simulink model "bus_14_take_1"  (Simulink 10.3)
settings: Solver=ode45  StartTime=0.0  StopTime=2  RelTol=1e-3
undefined symbols (not defined in the file): Discrete, linsys1, Time
libraries: spsThreePhaseVIMeasurementLib x46, spsThreePhasePISectionLineLib x20, spsThreePhaseSeriesRLCLoadLib x14, spsPMUPLLBasedPositiveSequenceLib x9, eePMU x5, spsThreePhaseTransformerTwoWindingsLib x5, spsPLLLib x4, ctrlSharedLib x3, spsSynchronousMachinepuStandardLib x3, spsThreePhaseParallelRLCLoadLib x3, spsThreePhaseBreakerLib x3, spsExcitationSystemLib x3
(part 1 of 2)
settings Model: Creator=User  LastModifiedBy=User
settings SolverCC: AlgebraicLoopSolver=Auto
settings DataIOCC: SaveFormat=Structure  SignalLoggingSaveFormat=Dataset  SaveOutput=off  SignalLogging=off  DSMLogging=off  SaveTime=off  ReturnWorkspaceOutputs=on  LoggingToFile=on
settings OptimizationCC: ExpressionDepthLimit=128  LifeSpan=auto  UseRowMajorAlgorithm=on
settings DebuggingCC: UnderspecifiedInitializationDetection=Simplified  MergeDetectMultiDrivingBlocksExec=error  FcnCallInpInsideContextMsg=error  StateNameClashWarn=none  SFUnexpectedBacktrackingDiag=error  SFNoUnconditionalDefaultTransitionDiag=error  SFExecutionAtInitializationDiag=warning  SFMachineParentedDataDiag=error  ArithmeticOperatorsInVariantConditions=error
settings HardwareCC: ProdBitPerPointer=64  ProdBitPerSizeT=64  ProdBitPerPtrDiffT=64  ProdLargestAtomicFloat=Float  ProdIntDivRoundTo=Zero  ProdEndianess=LittleEndian  ProdWordSize=64  ProdHWDeviceType=Intel->x86-64 (Windows64)
settings ModelReferenceCC: PropagateSignalLabelsOutOfModel=on
settings SFSimCC: SimUseLocalCustomCode=on  CustomCodeUndefinedFunction=FilterOut
settings RTWCC: RTWUseLocalCustomCode=on
settings CodeAppCC: StateflowObjectComments=off
settings GRTTargetCC: TargetLangStandard=C99 (ISO)  CombineOutputUpdateFcns=on  GRTInterface=off
settings ConfigComp: CovMetricSettings=dwe  CovSaveCumulativeToWorkspaceVar=off  CovSaveSingleToWorkspaceVar=off  CovExternalEMLEnable=on

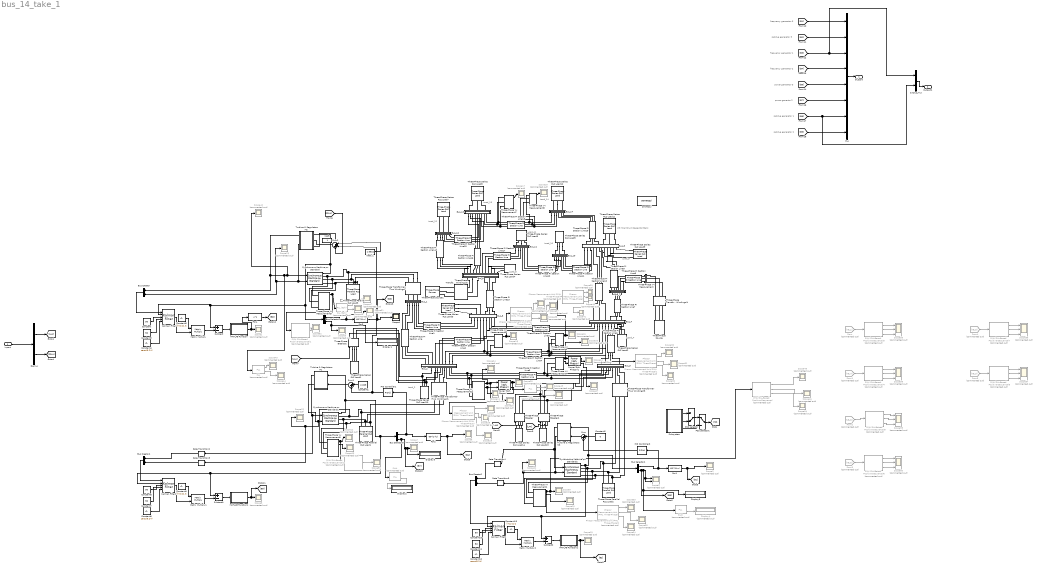
== system bus_14_take_1 ==
  note: residue generator 2
  note: residue generator 1
  note: power genertor 2
  note: power generator 3
  note: frequency generator 2
  note: frequency generator 1
  note: residue generator 3
  note: frequency generator 3
  note: Load_2
  note: Load_10
  note: Load_13
  note: Load_12
  note: 25 MVar Shunt
      | Capacitor Bank
  note: Load_9
  note: Load_11
  note: Load_6
  note: Load_4
  note: Load_14
  note: Load_5
  Inport : Inport
  Bus Creator : BusCreator  Inputs=2
  Bus Creator1 : BusCreator  Inputs=2
  Bus Creator2 : BusCreator  Inputs=2
  Bus Selector1 : BusSelector  OutputSignals="Mechanical.Rotor speed deviation  dw (pu),Mechanical.Electrical power  Pe (pu)"
  Bus Selector2 : BusSelector  OutputSignals="Mechanical.Rotor speed deviation  dw (pu),Mechanical.Electrical power  Pe (pu)"
  Bus Selector3 : BusSelector  OutputSignals="Mechanical.Rotor speed deviation  dw (pu),Mechanical.Electrical power  Pe (pu)"
  Bus_1 : Subsystem
  Bus_10 : Subsystem
  Bus_11 : Subsystem
  Bus_12 : Subsystem
  Bus_13 : Subsystem
  Bus_14 : Subsystem
  Bus_2 : Subsystem
  Bus_3 : Subsystem
  Bus_4 : Subsystem
  Bus_5 : Subsystem
  Bus_6 : Subsystem
  Bus_7 : Subsystem
  Bus_9 : Subsystem
  Constant{,3,6..7,10..11} (6 alike) : Constant  Value=50
  Constant1 : Constant  Value=2.009
  Constant12 : Constant  Value=zeros(8,24)
  Constant13 : Constant  Value=linsys1.C
  Constant2 : Constant  Value=0
  Constant4 : Constant  Value=zeros(8,24)
  Constant5 : Constant  Value=linsys1.C
  Constant8 : Constant  Value=zeros(8,24)
  Constant9 : Constant  Value=linsys1.C
  Demux : Demux  Outputs=2
  Display{1..3,5} (4 alike) : Display
  Display4 : Display  Commented=on
  Fcn1 : Fcn  Expr=60*(1+u)
  Fcn2 : Fcn  Expr=60*(1+u)
  Fcn3 : Fcn  Expr=60*(1+u)
  Fcn4 : Fcn  Expr=u*1
  From : From  Commented=on  GotoTag=VB_2  TagVisibility=global
  From1 : From  Commented=on  GotoTag=VB_4  TagVisibility=global
  From2 : From  Commented=on  GotoTag=VB_5  TagVisibility=global
  From3 : From  Commented=on  GotoTag=VB_6  TagVisibility=global
  From4 : From  Commented=on  GotoTag=VB_8  TagVisibility=global
  From5 : From  Commented=on  GotoTag=VB_9  TagVisibility=global
  Kalman Filter : ctrlSharedLib/Kalman Filter  TimeDomain=Discrete-Time  UseCurrentEstimator=on  ModelSource=Individual A, B, C, D matrices  ModelSourceVariable=ss(0.95,1,1,0,1)  A=linsys1.A  B=linsys1.B  C=linsys1.C  D=linsys1.D  NumberOfStates=1  NumberOfInputs=1  NumberOfOutputs=1  InitialEstimateSource=Dialog  X0=0  P0=10  UseK=off  UseGH=off  NumberOfProcessNoiseInputs=1  G=1  TimeInvariantG=on  H=0  TimeInvariantH=on  Q=0.05  TimeInvariantQ=off  R=1  TimeInvariantR=off  N=0  TimeInvariantN=off  AddInputPort=on  AddEnablePort=off  OutputEstimatedY=off  OutputP=off  Ts=-1
  Kalman Filter1 : ctrlSharedLib/Kalman Filter  TimeDomain=Discrete-Time  UseCurrentEstimator=on  ModelSource=Individual A, B, C, D matrices  ModelSourceVariable=ss(0.95,1,1,0,1)  A=linsys1.A  B=linsys1.B  C=linsys1.C  D=linsys1.D  NumberOfStates=1  NumberOfInputs=1  NumberOfOutputs=1  InitialEstimateSource=Dialog  X0=0  P0=10  UseK=off  UseGH=off  NumberOfProcessNoiseInputs=1  G=1  TimeInvariantG=on  H=0  TimeInvariantH=on  Q=0.05  TimeInvariantQ=off  R=1  TimeInvariantR=off  N=0  TimeInvariantN=off  AddInputPort=on  AddEnablePort=off  OutputEstimatedY=off  OutputP=off  Ts=-1
  Kalman Filter2 : ctrlSharedLib/Kalman Filter  TimeDomain=Discrete-Time  UseCurrentEstimator=on  ModelSource=Individual A, B, C, D matrices  ModelSourceVariable=ss(0.95,1,1,0,1)  A=linsys1.A  B=linsys1.B  C=linsys1.C  D=linsys1.D  NumberOfStates=1  NumberOfInputs=1  NumberOfOutputs=1  InitialEstimateSource=Dialog  X0=0  P0=10  UseK=off  UseGH=off  NumberOfProcessNoiseInputs=1  G=1  TimeInvariantG=on  H=0  TimeInvariantH=on  Q=0.05  TimeInvariantQ=off  R=1  TimeInvariantR=off  N=0  TimeInvariantN=off  AddInputPort=on  AddEnablePort=off  OutputEstimatedY=off  OutputP=off  Ts=-1
  MATLAB Function : MATLAB Function  TreatAsAtomicUnit=on
  MATLAB Function1 : MATLAB Function  TreatAsAtomicUnit=on
  MATLAB Function2 : MATLAB Function  TreatAsAtomicUnit=on
  Matrix Multiply : Product  Multiplication=Matrix(*)
  Matrix Multiply1 : Product  Multiplication=Matrix(*)
  Matrix Multiply2 : Product  Multiplication=Matrix(*)
  Mux : Mux  Inputs=8
  PID Controller1 : pid_lib/PID Controller  Controller=PID  Form=Parallel  TimeDomain=Discrete-time  UseExternalTs=off  SampleTime=-1  IntegratorMethod=Forward Euler  FilterMethod=Forward Euler  ControllerParametersSource=internal  P=-2.009  I=10  D=0  UseFilter=on  N=100  TunerSelectOption=Frequency Response Based  InitialConditionSource=internal  InitialConditionForIntegrator=0  InitialConditionForFilter=0  DifferentiatorICPrevScaledInput=0  ExternalReset=none  TrackingMode=off  Kt=1  LimitOutput=off  SatLimitsSource=internal  UpperSaturationLimit=inf  LowerSaturationLimit=-inf  LinearizeAsGain=on  AntiWindupMode=none  Kb=1  POutMin=[]  POutMax=[]  IOutMin=[]  IOutMax=[]  DOutMin=[]  DOutMax=[]  NOutMin=[]  NOutMax=[]  SumOutMin=[]  SumOutMax=[]  SaturationOutMin=[]  SaturationOutMax=[]  PParamMin=[]  PParamMax=[]  IParamMin=[]  IParamMax=[]  DParamMin=[]  DParamMax=[]  NParamMin=[]  NParamMax=[]  KbParamMin=[]  KbParamMax=[]  KtParamMin=[]  KtParamMax=[]  KbOutMin=[]  KbOutMax=[]  KtOutMin=[]  KtOutMax=[]  IntegratorOutMin=[]  IntegratorOutMax=[]  FilterOutMin=[]  FilterOutMax=[]  SumI1OutMin=[]  SumI1OutMax=[]  SumI2OutMin=[]  SumI2OutMax=[]  SumI3OutMin=[]  SumI3OutMax=[]  SumI4OutMin=[]  SumI4OutMax=[]  SumDOutMin=[]  SumDOutMax=[]  DifferentiatorOutMin=[]  DifferentiatorOutMax=[]  FilterDiffOutCoefMin=[]  FilterDiffOutCoefMax=[]  ReciprocalOutMin=[]  ReciprocalOutMax=[]  SumDenOutMin=[]  SumDenOutMax=[]  SumNumOutMin=[]  SumNumOutMax=[]  DivideOutMin=[]  DivideOutMax=[]  UdiffTsProdOutMin=[]  UdiffTsProdOutMax=[]  NTsProdOutMin=[]  NTsProdOutMax=[]  UintegralTsProdOutMin=[]  UintegralTsProdOutMax=[]  UngainTsProdOutMin=[]  UngainTsProdOutMax=[]  IntegratorContinuousStateAttributes=''  IntegratorStateMustResolveToSignalObject=off  IntegratorRTWStateStorageClass=Auto  FilterContinuousStateAttributes=''  FilterStateMustResolveToSignalObject=off  FilterRTWStateStorageClass=Auto  ParallelPVariant=InternalParameters  IdealPVariant=Disabled  IVariant=InternalParameters  DVariant=InternalParameters  IntegratorVariant=Discrete  SatVariant=Disabled  AWVariant=Passthrough  PCopyVariant=Disabled  TRVariant=Disabled  FdbkBlocksVariant=Forward  IdealPFdbkVariant=Disabled  SatFdbkVariant=Disabled  DerivativeFilterVariant=ForwardEulerFilter  NVariant=InternalParameters  NCopyVariant=Disabled  FilterICVariant=InternalICsFilter  IntegratorICVariant=InternalICs  ExternalResetVariant=Disabled  TRSumVariant=Passthrough  SumFdbkVariant=Disabled  SumVariant=Sum_PID  TsampFilterVariant=InternalTs  TsampNgainVariant=Passthrough  TsampIntegralVariant=Passthrough  ExternalSaturationOutDataTypeStr=Inherit: Same as second input
  PID Controller2 : pid_lib/PID Controller  Controller=PID  Form=Parallel  TimeDomain=Discrete-time  UseExternalTs=off  SampleTime=-1  IntegratorMethod=Forward Euler  FilterMethod=Forward Euler  ControllerParametersSource=internal  P=-2  I=10  D=0  UseFilter=on  N=100  TunerSelectOption=Transfer Function Based (PID Tuner App)  InitialConditionSource=internal  InitialConditionForIntegrator=0  InitialConditionForFilter=0  DifferentiatorICPrevScaledInput=0  ExternalReset=none  TrackingMode=off  Kt=1  LimitOutput=off  SatLimitsSource=internal  UpperSaturationLimit=inf  LowerSaturationLimit=-inf  LinearizeAsGain=on  AntiWindupMode=none  Kb=1  POutMin=[]  POutMax=[]  IOutMin=[]  IOutMax=[]  DOutMin=[]  DOutMax=[]  NOutMin=[]  NOutMax=[]  SumOutMin=[]  SumOutMax=[]  SaturationOutMin=[]  SaturationOutMax=[]  PParamMin=[]  PParamMax=[]  IParamMin=[]  IParamMax=[]  DParamMin=[]  DParamMax=[]  NParamMin=[]  NParamMax=[]  KbParamMin=[]  KbParamMax=[]  KtParamMin=[]  KtParamMax=[]  KbOutMin=[]  KbOutMax=[]  KtOutMin=[]  KtOutMax=[]  IntegratorOutMin=[]  IntegratorOutMax=[]  FilterOutMin=[]  FilterOutMax=[]  SumI1OutMin=[]  SumI1OutMax=[]  SumI2OutMin=[]  SumI2OutMax=[]  SumI3OutMin=[]  SumI3OutMax=[]  SumI4OutMin=[]  SumI4OutMax=[]  SumDOutMin=[]  SumDOutMax=[]  DifferentiatorOutMin=[]  DifferentiatorOutMax=[]  FilterDiffOutCoefMin=[]  FilterDiffOutCoefMax=[]  ReciprocalOutMin=[]  ReciprocalOutMax=[]  SumDenOutMin=[]  SumDenOutMax=[]  SumNumOutMin=[]  SumNumOutMax=[]  DivideOutMin=[]  DivideOutMax=[]  UdiffTsProdOutMin=[]  UdiffTsProdOutMax=[]  NTsProdOutMin=[]  NTsProdOutMax=[]  UintegralTsProdOutMin=[]  UintegralTsProdOutMax=[]  UngainTsProdOutMin=[]  UngainTsProdOutMax=[]  IntegratorContinuousStateAttributes=''  IntegratorStateMustResolveToSignalObject=off  IntegratorRTWStateStorageClass=Auto  FilterContinuousStateAttributes=''  FilterStateMustResolveToSignalObject=off  FilterRTWStateStorageClass=Auto  ParallelPVariant=InternalParameters  IdealPVariant=Disabled  IVariant=InternalParameters  DVariant=InternalParameters  IntegratorVariant=Discrete  SatVariant=Disabled  AWVariant=Passthrough  PCopyVariant=Disabled  TRVariant=Disabled  FdbkBlocksVariant=Forward  IdealPFdbkVariant=Disabled  SatFdbkVariant=Disabled  DerivativeFilterVariant=ForwardEulerFilter  NVariant=InternalParameters  NCopyVariant=Disabled  FilterICVariant=InternalICsFilter  IntegratorICVariant=InternalICs  ExternalResetVariant=Disabled  TRSumVariant=Passthrough  SumFdbkVariant=Disabled  SumVariant=Sum_PID  TsampFilterVariant=InternalTs  TsampNgainVariant=Passthrough  TsampIntegralVariant=Passthrough  ExternalSaturationOutDataTypeStr=Inherit: Same as second input
  PLL{,2,4..5} (4 alike) : spsPLLLib/PLL  Commented=on  Fmin=45  Par_Init=[0, 60]  ParK=[180, 3200, 1]  TcD=1e-4  MaxRateChangeFreq=12  FilterCutOffFreq=25  Ts=0  AGC=on
      settings: SourceProductBaseCode=PS
  PLL (3ph) : spsPLL3phLib/PLL (3ph)  Commented=on  Fmin=45  Par_Init=[0, 60]  ParK=[180, 3200, 1]  TcD=1e-4  MaxRateChangeFreq=12  FilterCutOffFreq=25  Ts=0  AGC=on
  PMU (PLL-Based, Positive-Sequence){,1..8} (9 alike) : spsPMUPLLBasedPositiveSequenceLib/PMU (PLL-Based, Positive-Sequence)  Commented=on  nominalFrequency=60  samplingRate=64  reportingFactor=1
      settings: SourceProductBaseCode=PS
  PSS selector : ManualSwitch  CurrentSetting=0
  PSS selector1 : ManualSwitch
  Phasor Measurement Unit (PMU, Three-Phase){,1..4} (5 alike) : eePMU/Phasor Measurement Unit (PMU, Three-Phase)  Commented=on  frequency=60  Nsr=64  k=1
      settings: SourceProductBaseCode=PS
  "Power (3ph, Phasor)" : spsPower3phPhasorLib/Power (3ph, Phasor)
      settings: SourceProductBaseCode=PS
  "Power (3ph, Phasor)1" : spsPower3phPhasorLib/Power (3ph, Phasor)
      settings: SourceProductBaseCode=PS
  Rate Transition{2..5} (4 alike) : RateTransition
  Scope{,1..2,5..54} (53 alike) : Scope  Commented=on
  Scope3 : Scope  Commented=on  NumInputPorts=2
  Scope4 : Scope
  Scope{55..60} (6 alike) : Scope  Commented=on  NumInputPorts=3
  Subsystem : Subsystem
  Subtract : Sum  Inputs=+-
  Subtract1 : Sum  Inputs=+-
  Subtract2 : Sum  Inputs=+-
  Sum : Sum  Inputs=|++
  Sum1 : Sum  Inputs=|++
  Sum2 : Sum  Inputs=|++-
  Synchronous Machine pu Standard : spsSynchronousMachinepuStandardLib/Synchronous Machine pu Standard  PresetModel=No  MechanicalLoad=Mechanical power Pm  ShowDetailedParameters=on  RotorType=Salient-pole  Units=per unit standard parameters  MeasurementBus=off  NominalParameters="[90E6  146280   60 ]"  Reactances1=[ 1.81, 0.3, 0.23, 1.76, 0.65, 0.25, 0.15 ]  Reactances2=[ 1.305, 0.296, 0.252, 0.474, 0.243, 0.18 ]  dAxisTimeConstants=Short-circuit  qAxisTimeConstants=Open-circuit  TimeConstants1="[ 4.4849  0.0681  0.1  ]"  TimeConstants2=[ 8.0, 0.03, 1.0, 0.07 ]  TimeConstants3="[  4.49  0.0681  0.0513  ]"  TimeConstants4=[ 8.0, 0.03, 0.3371, 0.0295 ]  TimeConstants5=[ 1.01, 0.053, 0.1 ]  TimeConstants6=[ 1.3201, 0.023, 1.0, 0.07 ]  TimeConstants7=[0.012 0.003 0.003]  TimeConstants8=[ 1.3201, 0.0231, 0.3371, 0.0295 ]  StatorResistance=2.8544e-3  Mechanical="[ 3.7 0  32]"  PolePairs=20  InitialConditions=[0 -55.1684 1.72023 1.72023 1.72023 -10.3587 -130.359 109.641 2.41694]  SetSaturation=off  Saturation=[0.6404,0.7127,0.8441,0.9214,0.9956,1.082,1.19,1.316,1.457;0.7,0.7698,0.8872,0.9466,0.9969,1.046,1.1,1.151,1.201]  LoadFlowParameters=[1 0 0 0 0]  TsPowergui=0  TsBlock=-1  IterativeModel=Trapezoidal non iterative  IterativeDiscreteModel=Trapezoidal non iterative  BusType=swing  Pref=0  Qref=0  Qmin=-inf  Qmax=inf  PLF=0  QLF=0
      settings: SourceProductBaseCode=PS
  Synchronous Machine pu Standard1 : spsSynchronousMachinepuStandardLib/Synchronous Machine pu Standard  PresetModel=No  MechanicalLoad=Mechanical power Pm  ShowDetailedParameters=on  RotorType=Salient-pole  Units=per unit standard parameters  MeasurementBus=off  NominalParameters="[90E6  144210   60 ]"  Reactances1=[ 1.81, 0.3, 0.23, 1.76, 0.65, 0.25, 0.15 ]  Reactances2=[ 1.305, 0.296, 0.252, 0.474, 0.243, 0.18 ]  dAxisTimeConstants=Short-circuit  qAxisTimeConstants=Open-circuit  TimeConstants1="[ 4.4849  0.0681  0.1  ]"  TimeConstants2=[ 8.0, 0.03, 1.0, 0.07 ]  TimeConstants3="[  4.49  0.0681  0.0513  ]"  TimeConstants4=[ 8.0, 0.03, 0.3371, 0.0295 ]  TimeConstants5=[ 1.01, 0.053, 0.1 ]  TimeConstants6=[ 1.3201, 0.023, 1.0, 0.07 ]  TimeConstants7=[0.012 0.003 0.003]  TimeConstants8=[ 1.3201, 0.0231, 0.3371, 0.0295 ]  StatorResistance=2.8544e-3  Mechanical="[ 3.7 0  32]"  PolePairs=20  InitialConditions=[0 -52.2742 2.06355 2.06355 2.06355 -13.2061 -133.206 106.794 2.88545]  SetSaturation=off  Saturation=[0.6404,0.7127,0.8441,0.9214,0.9956,1.082,1.19,1.316,1.457;0.7,0.7698,0.8872,0.9466,0.9969,1.046,1.1,1.151,1.201]  LoadFlowParameters=[1,0,0,0,0]  TsPowergui=0  TsBlock=-1  IterativeModel=Trapezoidal non iterative  IterativeDiscreteModel=Trapezoidal non iterative  BusType=PV  Pref=0  Qref=0  Qmin=-inf  Qmax=inf  PLF=0  QLF=0
      settings: SourceProductBaseCode=PS
  Synchronous Machine pu Standard2 : spsSynchronousMachinepuStandardLib/Synchronous Machine pu Standard  PresetModel=No  MechanicalLoad=Mechanical power Pm  ShowDetailedParameters=on  RotorType=Salient-pole  Units=per unit standard parameters  MeasurementBus=off  NominalParameters="[90E6  139380  60 ]"  Reactances1=[ 1.81, 0.3, 0.23, 1.76, 0.65, 0.25, 0.15 ]  Reactances2=[ 1.305, 0.296, 0.252, 0.474, 0.243, 0.18 ]  dAxisTimeConstants=Short-circuit  qAxisTimeConstants=Open-circuit  TimeConstants1="[ 4.4849  0.0681  0.1  ]"  TimeConstants2=[ 8.0, 0.03, 1.0, 0.07 ]  TimeConstants3="[  4.49  0.0681  0.0513  ]"  TimeConstants4=[ 8.0, 0.03, 0.3371, 0.0295 ]  TimeConstants5=[ 1.01, 0.053, 0.1 ]  TimeConstants6=[ 1.3201, 0.023, 1.0, 0.07 ]  TimeConstants7=[0.012 0.003 0.003]  TimeConstants8=[ 1.3201, 0.0231, 0.3371, 0.0295 ]  StatorResistance=2.8544e-3  Mechanical="[ 3.7 0  32]"  PolePairs=20  InitialConditions=[0 -114.329 0.550177 0.550177 0.550177 -114.259 -234.259 5.74123 1.7297]  SetSaturation=off  Saturation=[0.6404,0.7127,0.8441,0.9214,0.9956,1.082,1.19,1.316,1.457;0.7,0.7698,0.8872,0.9466,0.9969,1.046,1.1,1.151,1.201]  LoadFlowParameters=[1,0,0,0,0]  TsPowergui=0  TsBlock=-1  IterativeModel=Trapezoidal non iterative  IterativeDiscreteModel=Trapezoidal non iterative  BusType=PV  Pref=0  Qref=0  Qmin=50096006  Qmax=50096006  PLF=0  QLF=0
      settings: SourceProductBaseCode=PS
  Three-Phase PI Section Line : spsThreePhasePISectionLineLib/Three-Phase PI Section Line  LConnTagsString=a|b|c  RConnTagsString=A|B|C  Length=44.47  Frequency=60  Resistances=[ 0.1921 0.5763]  Inductances=[ 0.0016 0.0047]  Capacitances=[7.14e-9 2.14e-8]
  Three-Phase PI Section Line1 : spsThreePhasePISectionLineLib/Three-Phase PI Section Line  LConnTagsString=a|b|c  RConnTagsString=A|B|C  Length=78.64  Frequency=60  Resistances=[ 0.3029 0.9086]  Inductances=[ 0.0033 0.0099]  Capacitances=[3.35e-9 1.01e-8]
  Three-Phase PI Section Line10 : spsThreePhasePISectionLineLib/Three-Phase PI Section Line  LConnTagsString=a|b|c  RConnTagsString=A|B|C  Length=8.39  Frequency=60  Resistances=[ 0.0001 0.0003]  Inductances=[ 0.0775 0.2325]  Capacitances=[1.43e-10 4.3e-10]
  Three-Phase PI Section Line11 : spsThreePhasePISectionLineLib/Three-Phase PI Section Line  LConnTagsString=a|b|c  RConnTagsString=A|B|C  Length=3.27  Frequency=60  Resistances=[ 0.2144 0.6431]  Inductances=[ 0.0015 0.0045]  Capacitances=[1.84e-11 5.52e-11]
  Three-Phase PI Section Line12 : spsThreePhasePISectionLineLib/Three-Phase PI Section Line  LConnTagsString=a|b|c  RConnTagsString=A|B|C  Length=4.93  Frequency=60  Resistances=[ 0.3667 1.1002]  Inductances=[ 0.0023 0.0068]  Capacitances=[1.22e-11 3.66e-11]
  Three-Phase PI Section Line13 : spsThreePhasePISectionLineLib/Three-Phase PI Section Line  LConnTagsString=a|b|c  RConnTagsString=A|B|C  Length=5.65  Frequency=60  Resistances=[ 0.0001 0.0003]  Inductances=[ 0.0522 0.1565]  Capacitances=[2.13e-10 6.39e-10]
  Three-Phase PI Section Line14 : spsThreePhasePISectionLineLib/Three-Phase PI Section Line  LConnTagsString=a|b|c  RConnTagsString=A|B|C  Length=5.69  Frequency=60  Resistances=[ 0.4760 1.4281]  Inductances=[ 0.0026 0.0079]  Capacitances=[1.06e-11 3.17e-11]
  Three-Phase PI Section Line15 : spsThreePhasePISectionLineLib/Three-Phase PI Section Line  LConnTagsString=a|b|c  RConnTagsString=A|B|C  Length=5.03  Frequency=60  Resistances=[ 0.9679 2.9038]  Inductances=[ 0.0023 0.0070]  Capacitances=[1.20e-11 3.59e-11]
  Three-Phase PI Section Line16 : spsThreePhasePISectionLineLib/Three-Phase PI Section Line  LConnTagsString=a|b|c  RConnTagsString=A|B|C  Length=4.06  Frequency=60  Resistances=[ 0.3590 1.0770]  Inductances=[ 0.0019 0.0056]  Capacitances=[1.48e-11 4.44e-11]
  Three-Phase PI Section Line17 : spsThreePhasePISectionLineLib/Three-Phase PI Section Line  LConnTagsString=a|b|c  RConnTagsString=A|B|C  Length=5.02  Frequency=60  Resistances=[ 0.4172 1.2515]  Inductances=[ 0.0023 0.0070]  Capacitances=[1.20e-11 3.60e-11]
  Three-Phase PI Section Line18 : spsThreePhasePISectionLineLib/Three-Phase PI Section Line  LConnTagsString=a|b|c  RConnTagsString=A|B|C  Length=6.64  Frequency=60  Resistances=[ 0.5676 1.7027]  Inductances=[ 0.0031 0.0092]  Capacitances=[9.06e-12 2.72e-11]
  Three-Phase PI Section Line19 : spsThreePhasePISectionLineLib/Three-Phase PI Section Line  LConnTagsString=a|b|c  RConnTagsString=A|B|C  Length=5.85  Frequency=60  Resistances=[ 0.4788 1.4365]  Inductances=[ 0.0027 0.0081]  Capacitances=[1.03e-11 3.08e-11]
  Three-Phase PI Section Line2 : spsThreePhasePISectionLineLib/Three-Phase PI Section Line  LConnTagsString=a|b|c  RConnTagsString=A|B|C  Length=61.18  Frequency=60  Resistances=[ 0.4104 1.2311]  Inductances=[ 0.0033 0.0100]  Capacitances=[3.34e-9 1.0e-8]
  Three-Phase PI Section Line3 : spsThreePhasePISectionLineLib/Three-Phase PI Section Line  LConnTagsString=a|b|c  RConnTagsString=A|B|C  Length=18.47  Frequency=60  Resistances=[ 0.3186 0.9558]  Inductances=[ 0.0027 0.0080]  Capacitances=[4.17e-9 1.25e-8]
  Three-Phase PI Section Line4 : spsThreePhasePISectionLineLib/Three-Phase PI Section Line  LConnTagsString=a|b|c  RConnTagsString=A|B|C  Length=74.11  Frequency=60  Resistances=[ 0.3457 1.0370]  Inductances=[ 0.0028 0.0083]  Capacitances=[3.99e-9 1.20e-8]
  Three-Phase PI Section Line5 : spsThreePhasePISectionLineLib/Three-Phase PI Section Line  LConnTagsString=a|b|c  RConnTagsString=A|B|C  Length=68.47  Frequency=60  Resistances=[ 0.3026 0.9077]  Inductances=[ 0.0034 0.0101]  Capacitances=[3.29e-9 9.86e-8]
  Three-Phase PI Section Line6 : spsThreePhasePISectionLineLib/Three-Phase PI Section Line  LConnTagsString=a|b|c  RConnTagsString=A|B|C  Length=61.21  Frequency=60  Resistances=[ 0.4826 1.4479]  Inductances=[ 0.0033 0.0098]  Capacitances=[3.4e-9 1.02e-8]
  Three-Phase PI Section Line7 : spsThreePhasePISectionLineLib/Three-Phase PI Section Line  LConnTagsString=a|b|c  RConnTagsString=A|B|C  Length=5.15  Frequency=60  Resistances=[ 0.0001 0.0003]  Inductances=[ 0.0475 0.1425]  Capacitances=[2.34e-10 7.02e-10]
  Three-Phase PI Section Line8 : spsThreePhasePISectionLineLib/Three-Phase PI Section Line  LConnTagsString=a|b|c  RConnTagsString=A|B|C  Length=4.72  Frequency=60  Resistances=[ 0.0005 0.0014]  Inductances=[ 0.0022 0.0065]  Capacitances=[ 1.27e-11 3.82e-11]
  Three-Phase PI Section Line9 : spsThreePhasePISectionLineLib/Three-Phase PI Section Line  LConnTagsString=a|b|c  RConnTagsString=A|B|C  Length=3.73  Frequency=60  Resistances=[ 0.0006 0.0018]  Inductances=[ 0.0017 0.0052]  Capacitances=[ 1.61e-11 4.84e-11]
  Three-Phase Parallel RLC Load1 : spsThreePhaseParallelRLCLoadLib/Three-Phase Parallel RLC Load  LConnTagsString=A|B|C  Configuration=Y (grounded)  NominalVoltage=10000  Vabc=[1e3 1e3 1e3]  Vabcp=[1e3 1e3 1e3]  NominalFrequency=60  UnbalancedPower=off  ActivePower=10e3  InductivePower=2000  CapacitivePower=0  Pabc=[10e3 9e3 11e3]  QLabc=[100 90 110]  QCabc=[100 90 110]  Pabcp=[10e3 9e3 11e3]  QLabcp=[100 90 110]  QCabcp=[100 90 110]  Measurements=None  LoadType=constant Z
  Three-Phase Parallel RLC Load2 : spsThreePhaseParallelRLCLoadLib/Three-Phase Parallel RLC Load  LConnTagsString=A|B|C  Configuration=Y (grounded)  NominalVoltage=10000  Vabc=[1e3 1e3 1e3]  Vabcp=[1e3 1e3 1e3]  NominalFrequency=60  UnbalancedPower=off  ActivePower=10e3  InductivePower=2000  CapacitivePower=0  Pabc=[10e3 9e3 11e3]  QLabc=[100 90 110]  QCabc=[100 90 110]  Pabcp=[10e3 9e3 11e3]  QLabcp=[100 90 110]  QCabcp=[100 90 110]  Measurements=None  LoadType=constant Z
  Three-Phase Parallel RLC Load3 : spsThreePhaseParallelRLCLoadLib/Three-Phase Parallel RLC Load  LConnTagsString=A|B|C  Configuration=Y (grounded)  NominalVoltage=10000  Vabc=[1e3 1e3 1e3]  Vabcp=[1e3 1e3 1e3]  NominalFrequency=60  UnbalancedPower=off  ActivePower=10e3  InductivePower=2000  CapacitivePower=0  Pabc=[10e3 9e3 11e3]  QLabc=[100 90 110]  QCabc=[100 90 110]  Pabcp=[10e3 9e3 11e3]  QLabcp=[100 90 110]  QCabcp=[100 90 110]  Measurements=None  LoadType=constant Z
  Three-Phase Series RLC Load1 : spsThreePhaseSeriesRLCLoadLib/Three-Phase Series RLC Load  LConnTagsString=A|B|C  Configuration=Y (grounded)  NominalVoltage=(217684)*1  Vabc=[1e3 1e3 1e3]  Vabcp=[1e3 1e3 1e3]  NominalFrequency=60  UnbalancedPower=off  ActivePower=1130400000000  InductivePower=228000000000  CapacitivePower=0  Pabc=[10e3 9e3 11e3]  QLabc=[100 90 110]  QCabc=[100 90 110]  Pabcp=[10e3 9e3 11e3]  QLabcp=[100 90 110]  QCabcp=[100 90 110]  Measurements=None  LoadType=constant PQ
  Three-Phase Series RLC Load10 : spsThreePhaseSeriesRLCLoadLib/Three-Phase Series RLC Load  LConnTagsString=A|B|C  Configuration=Y (grounded)  NominalVoltage=(222552)*1  Vabc=[1e3 1e3 1e3]  Vabcp=[1e3 1e3 1e3]  NominalFrequency=60  UnbalancedPower=off  ActivePower=26040000  InductivePower=15240000  CapacitivePower=0  Pabc=[10e3 9e3 11e3]  QLabc=[100 90 110]  QCabc=[100 90 110]  Pabcp=[10e3 9e3 11e3]  QLabcp=[100 90 110]  QCabcp=[100 90 110]  Measurements=None  LoadType=constant PQ
  Three-Phase Series RLC Load11 : spsThreePhaseSeriesRLCLoadLib/Three-Phase Series RLC Load  LConnTagsString=A|B|C  Configuration=Y (grounded)  NominalVoltage=230e3  Vabc=[1e3 1e3 1e3]  Vabcp=[1e3 1e3 1e3]  NominalFrequency=60  UnbalancedPower=off  ActivePower=0  InductivePower=0  CapacitivePower=25000000  Pabc=[10e3 9e3 11e3]  QLabc=[100 90 110]  QCabc=[100 90 110]  Pabcp=[10e3 9e3 11e3]  QLabcp=[100 90 110]  QCabcp=[100 90 110]  Measurements=None  LoadType=constant Z
  Three-Phase Series RLC Load12 : spsThreePhaseSeriesRLCLoadLib/Three-Phase Series RLC Load  LConnTagsString=A|B|C  Configuration=Y (grounded)  NominalVoltage=(221100)*1  Vabc=[1e3 1e3 1e3]  Vabcp=[1e3 1e3 1e3]  NominalFrequency=60  UnbalancedPower=off  ActivePower=17880000  InductivePower=6000000  CapacitivePower=0  Pabc=[10e3 9e3 11e3]  QLabc=[100 90 110]  QCabc=[100 90 110]  Pabcp=[10e3 9e3 11e3]  QLabcp=[100 90 110]  QCabcp=[100 90 110]  Measurements=None  LoadType=constant PQ
  Three-Phase Series RLC Load13 : spsThreePhaseSeriesRLCLoadLib/Three-Phase Series RLC Load  LConnTagsString=A|B|C  Configuration=Y (grounded)  NominalVoltage=(217684)*1  Vabc=[1e3 1e3 1e3]  Vabcp=[1e3 1e3 1e3]  NominalFrequency=60  UnbalancedPower=off  ActivePower=113040000  InductivePower=22800000  CapacitivePower=0  Pabc=[10e3 9e3 11e3]  QLabc=[100 90 110]  QCabc=[100 90 110]  Pabcp=[10e3 9e3 11e3]  QLabcp=[100 90 110]  QCabcp=[100 90 110]  Measurements=None  LoadType=constant PQ
  Three-Phase Series RLC Load14 : spsThreePhaseSeriesRLCLoadLib/Three-Phase Series RLC Load  LConnTagsString=A|B|C  Configuration=Y (grounded)  NominalVoltage=(217684)*1  Vabc=[1e3 1e3 1e3]  Vabcp=[1e3 1e3 1e3]  NominalFrequency=60  UnbalancedPower=off  ActivePower=1130400000000  InductivePower=228000000000  CapacitivePower=0  Pabc=[10e3 9e3 11e3]  QLabc=[100 90 110]  QCabc=[100 90 110]  Pabcp=[10e3 9e3 11e3]  QLabcp=[100 90 110]  QCabcp=[100 90 110]  Measurements=None  LoadType=constant PQ
  Three-Phase Series RLC Load2 : spsThreePhaseSeriesRLCLoadLib/Three-Phase Series RLC Load  LConnTagsString=A|B|C  Configuration=Y (grounded)  NominalVoltage=(217810)*1  Vabc=[1e3 1e3 1e3]  Vabcp=[1e3 1e3 1e3]  NominalFrequency=60  UnbalancedPower=off  ActivePower=57360000  InductivePower=0  CapacitivePower=4680000  Pabc=[10e3 9e3 11e3]  QLabc=[100 90 110]  QCabc=[100 90 110]  Pabcp=[10e3 9e3 11e3]  QLabcp=[100 90 110]  QCabcp=[100 90 110]  Measurements=None  LoadType=constant PQ
  Three-Phase Series RLC Load3 : spsThreePhaseSeriesRLCLoadLib/Three-Phase Series RLC Load  LConnTagsString=A|B|C  Configuration=Y (grounded)  NominalVoltage=(218590)*1  Vabc=[1e3 1e3 1e3]  Vabcp=[1e3 1e3 1e3]  NominalFrequency=60  UnbalancedPower=off  ActivePower=9120000  InductivePower=1920000  CapacitivePower=0  Pabc=[10e3 9e3 11e3]  QLabc=[100 90 110]  QCabc=[100 90 110]  Pabcp=[10e3 9e3 11e3]  QLabcp=[100 90 110]  QCabcp=[100 90 110]  Measurements=None  LoadType=constant PQ
  Three-Phase Series RLC Load4 : spsThreePhaseSeriesRLCLoadLib/Three-Phase Series RLC Load  LConnTagsString=A|B|C  Configuration=Y (grounded)  NominalVoltage=(221344)*1.00001  Vabc=[1e3 1e3 1e3]  Vabcp=[1e3 1e3 1e3]  NominalFrequency=60  UnbalancedPower=off  ActivePower=13440000  InductivePower=9000000  CapacitivePower=0  Pabc=[10e3 9e3 11e3]  QLabc=[100 90 110]  QCabc=[100 90 110]  Pabcp=[10e3 9e3 11e3]  QLabcp=[100 90 110]  QCabcp=[100 90 110]  Measurements=None  LoadType=constant PQ
  Three-Phase Series RLC Load5 : spsThreePhaseSeriesRLCLoadLib/Three-Phase Series RLC Load  LConnTagsString=A|B|C  Configuration=Y (grounded)  NominalVoltage=(221346)*1  Vabc=[1e3 1e3 1e3]  Vabcp=[1e3 1e3 1e3]  NominalFrequency=60  UnbalancedPower=off  ActivePower=10800000  InductivePower=6960000  CapacitivePower=0  Pabc=[10e3 9e3 11e3]  QLabc=[100 90 110]  QCabc=[100 90 110]  Pabcp=[10e3 9e3 11e3]  QLabcp=[100 90 110]  QCabcp=[100 90 110]  Measurements=None  LoadType=constant PQ
  Three-Phase Series RLC Load6 : spsThreePhaseSeriesRLCLoadLib/Three-Phase Series RLC Load  LConnTagsString=A|B|C  Configuration=Y (grounded)  NominalVoltage=(221304)*1  Vabc=[1e3 1e3 1e3]  Vabcp=[1e3 1e3 1e3]  NominalFrequency=60  UnbalancedPower=off  ActivePower=4200000  InductivePower=2160000  CapacitivePower=0  Pabc=[10e3 9e3 11e3]  QLabc=[100 90 110]  QCabc=[100 90 110]  Pabcp=[10e3 9e3 11e3]  QLabcp=[100 90 110]  QCabcp=[100 90 110]  Measurements=None  LoadType=constant PQ
  Three-Phase Series RLC Load7 : spsThreePhaseSeriesRLCLoadLib/Three-Phase Series RLC Load  LConnTagsString=A|B|C  Configuration=Y (grounded)  NominalVoltage=(221181)*1  Vabc=[1e3 1e3 1e3]  Vabcp=[1e3 1e3 1e3]  NominalFrequency=60  UnbalancedPower=off  ActivePower=7320000  InductivePower=1920000  CapacitivePower=0  Pabc=[10e3 9e3 11e3]  QLabc=[100 90 110]  QCabc=[100 90 110]  Pabcp=[10e3 9e3 11e3]  QLabcp=[100 90 110]  QCabcp=[100 90 110]  Measurements=None  LoadType=constant PQ
  Three-Phase Series RLC Load8 : spsThreePhaseSeriesRLCLoadLib/Three-Phase Series RLC Load  LConnTagsString=A|B|C  Configuration=Y (grounded)  NominalVoltage=(221144)*0.999998  Vabc=[1e3 1e3 1e3]  Vabcp=[1e3 1e3 1e3]  NominalFrequency=60  UnbalancedPower=off  ActivePower=16200000  InductivePower=6960000  CapacitivePower=0  Pabc=[10e3 9e3 11e3]  QLabc=[100 90 110]  QCabc=[100 90 110]  Pabcp=[10e3 9e3 11e3]  QLabcp=[100 90 110]  QCabcp=[100 90 110]  Measurements=None  LoadType=constant PQ
  Three-Phase Series RLC Load9 : spsThreePhaseSeriesRLCLoadLib/Three-Phase Series RLC Load  LConnTagsString=A|B|C  Configuration=Y (grounded)  NominalVoltage=(221458)*1  Vabc=[1e3 1e3 1e3]  Vabcp=[1e3 1e3 1e3]  NominalFrequency=60  UnbalancedPower=off  ActivePower=35400000  InductivePower=19920000  CapacitivePower=0  Pabc=[10e3 9e3 11e3]  QLabc=[100 90 110]  QCabc=[100 90 110]  Pabcp=[10e3 9e3 11e3]  QLabcp=[100 90 110]  QCabcp=[100 90 110]  Measurements=None  LoadType=constant PQ
  Three-Phase Transformer (Two Windings) : spsThreePhaseTransformerTwoWindingsLib/Three-Phase Transformer (Two Windings)  Winding1Connection=Yg  Winding2Connection=Yg  CoreType=Three single-phase transformers  SetSaturation=off  Hysteresis=off  DataFile='hysteresis'  SetInitialFlux=off  Measurements=None  UNITS=pu  NominalPower=[ 120e6 , 60 ]  Winding1=[146.28e3 , 0.002 , 0.08 ]  Winding2=[ 230e3 , 0.002 , 0.08 ]  Rm=500  Lm=500  L0=0.5  Saturation=[ 0,0 ; 0.0024,1.2 ; 1.0,1.52 ]  InitialFluxes=[ 0.8 , -0.8 , 0.7 ]  BreakLoop=off  DiscreteSolver=Trapezoidal iterative  DataType=off  TransfoNumber=1
  Three-Phase Transformer (Two Windings)1 : spsThreePhaseTransformerTwoWindingsLib/Three-Phase Transformer (Two Windings)  Winding1Connection=Yg  Winding2Connection=Yg  CoreType=Three single-phase transformers  SetSaturation=off  Hysteresis=off  DataFile='hysteresis'  SetInitialFlux=off  Measurements=None  UNITS=pu  NominalPower=[ 120e6 , 60 ]  Winding1=[144.21e3 , 0.002 , 0.08 ]  Winding2=[ 230e3 , 0.002 , 0.08 ]  Rm=500  Lm=500  L0=0.5  Saturation=[ 0,0 ; 0.0024,1.2 ; 1.0,1.52 ]  InitialFluxes=[ 0.8 , -0.8 , 0.7 ]  BreakLoop=off  DiscreteSolver=Trapezoidal iterative  DataType=off  TransfoNumber=1
  Three-Phase Transformer (Two Windings)2 : spsThreePhaseTransformerTwoWindingsLib/Three-Phase Transformer (Two Windings)  Winding1Connection=Yg  Winding2Connection=Yg  CoreType=Three single-phase transformers  SetSaturation=off  Hysteresis=off  DataFile='hysteresis'  SetInitialFlux=off  Measurements=None  UNITS=pu  NominalPower=[ 120e6 , 60 ]  Winding1=[147.66e3 , 0.002 , 0.08 ]  Winding2=[ 230e3 , 0.002 , 0.08 ]  Rm=500  Lm=500  L0=0.5  Saturation=[ 0,0 ; 0.0024,1.2 ; 1.0,1.52 ]  InitialFluxes=[ 0.8 , -0.8 , 0.7 ]  BreakLoop=off  DiscreteSolver=Trapezoidal iterative  DataType=off  TransfoNumber=1
  Three-Phase Transformer (Two Windings)3 : spsThreePhaseTransformerTwoWindingsLib/Three-Phase Transformer (Two Windings)  Winding1Connection=Yg  Winding2Connection=Yg  CoreType=Three single-phase transformers  SetSaturation=off  Hysteresis=off  DataFile='hysteresis'  SetInitialFlux=off  Measurements=None  UNITS=pu  NominalPower=[ 120e6 , 60 ]  Winding1=[139.38e3 , 0.002 , 0.08 ]  Winding2=[ 230e3 , 0.002 , 0.08 ]  Rm=500  Lm=500  L0=0.5  Saturation=[ 0,0 ; 0.0024,1.2 ; 1.0,1.52 ]  InitialFluxes=[ 0.8 , -0.8 , 0.7 ]  BreakLoop=off  DiscreteSolver=Trapezoidal iterative  DataType=off  TransfoNumber=1
  Three-Phase Transformer (Two Windings)4 : spsThreePhaseTransformerTwoWindingsLib/Three-Phase Transformer (Two Windings)  Winding1Connection=Yg  Winding2Connection=Yg  CoreType=Three single-phase transformers  SetSaturation=off  Hysteresis=off  DataFile='hysteresis'  SetInitialFlux=off  Measurements=None  UNITS=pu  NominalPower=[ 120e6 , 60 ]  Winding1=[150.42e3 , 0.002 , 0.08 ]  Winding2=[ 230e3 , 0.002 , 0.08 ]  Rm=500  Lm=500  L0=0.5  Saturation=[ 0,0 ; 0.0024,1.2 ; 1.0,1.52 ]  InitialFluxes=[ 0.8 , -0.8 , 0.7 ]  BreakLoop=off  DiscreteSolver=Trapezoidal iterative  DataType=off  TransfoNumber=1
  Three-Phase V-I Measurement : spsThreePhaseVIMeasurementLib/Three-Phase V-I Measurement  VoltageMeasurement=phase-to-phase  SetLabelV=on  LabelV=VB_8  Vpu=off  VpuLL=off  CurrentMeasurement=yes  SetLabelI=on  LabelI=IB_8  Ipu=off  Pbase=100e6  Vbase=500e3  OutputType=Complex  PhasorSimulation=off  PSBequivalent=0
  Three-Phase V-I Measurement{1..9} (9 alike) : spsThreePhaseVIMeasurementLib/Three-Phase V-I Measurement  VoltageMeasurement=phase-to-ground  SetLabelV=off  LabelV=Vabc  Vpu=off  VpuLL=off  CurrentMeasurement=yes  SetLabelI=off  LabelI=Iabc  Ipu=off  Pbase=100e6  Vbase=500e3  OutputType=Complex  PhasorSimulation=off  PSBequivalent=0
  Three-Phase Breaker : spsThreePhaseBreakerLib/Three-Phase Breaker  InitialState=open  SwitchA=on  SwitchB=on  SwitchC=on  SwitchTimes=[0.1 0.9]  External=on  BreakerResistance=0.01  SnubberResistance=1e6  SnubberCapacitance=inf  Measurements=None
  Three-Phase Breaker1 : spsThreePhaseBreakerLib/Three-Phase Breaker  InitialState=open  SwitchA=on  SwitchB=on  SwitchC=on  SwitchTimes=[0.1 0.9]  External=on  BreakerResistance=0.01  SnubberResistance=1e6  SnubberCapacitance=inf  Measurements=None
  Three-Phase Breaker2 : spsThreePhaseBreakerLib/Three-Phase Breaker  InitialState=open  SwitchA=on  SwitchB=on  SwitchC=on  SwitchTimes=[0.1 0.9]  External=on  BreakerResistance=0.01  SnubberResistance=1e6  SnubberCapacitance=inf  Measurements=None
  Three-Phase Source : spsThreePhaseSourceLib/Three-Phase Source  InternalConnection=Yg  VoltagePhases=off  Voltage=(150420)*1.01398  PhaseAngle=-26.0476  Voltage_phases=[25e3 25e3 25e3]/sqrt(3)  PhaseAngles_phases=[0 -120 +120]  Frequency=60  NonIdealSource=on  SpecifyImpedance=off  Resistance=0.8929  Inductance=16.58e-3  ShortCircuitLevel=100e6  BaseVoltage=150.42e3  XRratio=7  BusType=PQ  Pref=0  Qref=30144000  Prefabc=[10e3, 10e3, 10e3]  Qrefabc=[0, 0, 0]  Qmin=-inf  Qmax=inf
  Three-Phase Source1 : spsThreePhaseSourceLib/Three-Phase Source  InternalConnection=Yg  VoltagePhases=off  Voltage=(147660)*1.00332  PhaseAngle=-26.1108  Voltage_phases=[25e3 25e3 25e3]/sqrt(3)  PhaseAngles_phases=[0 -120 +120]  Frequency=60  NonIdealSource=on  SpecifyImpedance=off  Resistance=0.8929  Inductance=16.58e-3  ShortCircuitLevel=100e6  BaseVoltage=147.66e3  XRratio=7  BusType=PQ  Pref=0  Qref=25276000  Prefabc=[10e3, 10e3, 10e3]  Qrefabc=[0, 0, 0]  Qmin=-inf  Qmax=inf
  Turbine & Regulators M1 : Subsystem
  Turbine & Regulators M2 : Subsystem
  Turbine & Regulators M3 : Subsystem
  Vref1 1 : Constant  Value=1.6922
  Vref2 : Constant
  output_mux : Mux  Inputs=2
  powergui : spspowerguiLib/powergui  Priority=1  SimulationMode=Discrete  SampleTime=50e-6  frequency=60  Iterations=2000  frequencyindice=60  Pbase=100e6  ErrMax=0.0001  UnitsV=kV  UnitsW=MW  buscounter=0  FunctionMessages=off  echomessages=off  EnableUseOfTLC=off  CurrentSourceSwitches=off  DisableSnubberDevices=off  DisableRonSwitches=off  DisableVfSwitches=off  DisplayEquations=off  AutomaticDiscreteSolvers=off  SolverType=Tustin/Backward Euler (TBE)  Interpol=off  ExternalGateDelay=off  methode=off  Ts=100  x0status=blocks  SPID=on  SwTol=0  HookPort=off  NonlinearTolerance=1e-4  nMaxIteration=100  ContinueOnMaxIteration=off  RestoreLinks=warning  ResistiveCurrentMeasurement=off  Frange=[0:2:500]  Ylog=off  Xlog=on  ShowGrid=off  save=off  variable=ZData  structure=0  ZoomFFT=off  StartTime=0.0  cycles=1  DisplayStyle=1  fundamental=60  FreqAxis=off  MaxFrequency=1000  frequencyindicesteady=1  RmsSteady=1  display=off
  Outport : Outport
  Outport1 : Outport  Port=2
  tag scope: PSS=global
  wires:
  "PMU (PLL-Based, Positive-Sequence)4"/2 -> Scope58/2
  "PMU (PLL-Based, Positive-Sequence)1"/2 -> Scope52/1
  Rate Transition4/1 -> Bus Creator2/1
  "PMU (PLL-Based, Positive-Sequence)7"/3 -> Scope56/3
  Constant12/1 -> Kalman Filter2/5
  "PMU (PLL-Based, Positive-Sequence)6"/2 -> Scope60/2
  From/1 -> "PMU (PLL-Based, Positive-Sequence)3"/1
  "PMU (PLL-Based, Positive-Sequence)3"/2 -> Scope55/2
  "PMU (PLL-Based, Positive-Sequence)6"/1 -> Scope60/1
  "Phasor Measurement Unit (PMU, Three-Phase)4"/2 -> Scope40/1
  PLL2/2 -> Scope50/1
  From4/1 -> "PMU (PLL-Based, Positive-Sequence)7"/1
  "PMU (PLL-Based, Positive-Sequence)7"/2 -> Scope56/2
  "PMU (PLL-Based, Positive-Sequence)4"/3 -> Scope58/3
  "Phasor Measurement Unit (PMU, Three-Phase)3"/2 -> Scope37/1
  "Power (3ph, Phasor)1"/2 -> Scope27/1
  Three-Phase V-I Measurement4/2 -> "Power (3ph, Phasor)1"/2
  PLL5/2 -> Display4/1
  From1/1 -> "PMU (PLL-Based, Positive-Sequence)4"/1
  "PMU (PLL-Based, Positive-Sequence)5"/2 -> Scope59/2
  Turbine & Regulators M2/1(Pm) -> PLL/1, Scope42/1, Synchronous Machine pu Standard/1, Bus Creator/1
  "Phasor Measurement Unit (PMU, Three-Phase)1"/1 -> Scope30/1
  [LAA] -> Three-Phase Breaker/1
  "PMU (PLL-Based, Positive-Sequence)5"/3 -> Scope59/3
  PLL/2 -> Scope44/1
  Rate Transition3/1 -> Bus Creator1/2
  "PMU (PLL-Based, Positive-Sequence)"/1 -> Scope45/1
  Rate Transition5/1 -> Bus Creator2/2
  "Phasor Measurement Unit (PMU, Three-Phase)4"/3 -> Scope41/1
  Subsystem/1(Generic) -> PSS selector/1
  Bus Creator/1 -> Kalman Filter/1
  Bus Creator2/1 -> Kalman Filter2/1
  "PMU (PLL-Based, Positive-Sequence)"/2 -> Scope46/1
  Subsystem/3(No PSS) -> PSS selector1/2
  PLL2/1 -> Scope49/1
  PLL (3ph)/2 -> Scope48/1
  Subsystem/2(Multiband) -> PSS selector/2
  Three-Phase V-I Measurement9/1 -> "PMU (PLL-Based, Positive-Sequence)1"/1, PLL (3ph)/1
  "Power (3ph, Phasor)"/2 -> Scope26/1
  Constant10/1 -> Kalman Filter2/3
  [LAA] -> Three-Phase Breaker1/1
  Subtract2/1 -> MATLAB Function2/1(u)
  Matrix Multiply2/1 -> Subtract2/2
  "PMU (PLL-Based, Positive-Sequence)8"/2 -> Scope57/2
  Three-Phase V-I Measurement2/2 -> Scope11/1, "Power (3ph, Phasor)"/2
  From5/1 -> "PMU (PLL-Based, Positive-Sequence)8"/1
  Three-Phase V-I Measurement1/1 -> "Phasor Measurement Unit (PMU, Three-Phase)2"/1, "PMU (PLL-Based, Positive-Sequence)"/1, Scope9/1
  Sum1/1 -> Turbine & Regulators M1/2(Pref)
  Three-Phase V-I Measurement2/1 -> Scope24/1, "Phasor Measurement Unit (PMU, Three-Phase)"/1, "Power (3ph, Phasor)"/1
  "PMU (PLL-Based, Positive-Sequence)"/3 -> Scope54/1
  Constant13/1 -> Matrix Multiply2/1
  Bus Creator1/1 -> Kalman Filter1/1
  Constant8/1 -> Kalman Filter1/5
  Constant3/1 -> Kalman Filter/4
  Three-Phase V-I Measurement1/2 -> Scope10/1
  Sum/1 -> Turbine & Regulators M3/2(Pref)
  Three-Phase V-I Measurement6/1 -> "Phasor Measurement Unit (PMU, Three-Phase)4"/1, Scope16/1
  Kalman Filter/1 -> Matrix Multiply/2
  [LAA] -> Three-Phase Breaker2/1
  MATLAB Function/1(y) -> Fcn4/1, Scope1/1
  Vref2/1 -> Turbine & Regulators M2/3(Vref)
  Constant/1 -> Kalman Filter/3
  Subtract1/1 -> MATLAB Function1/1(u)
  Sum2/1 -> Turbine & Regulators M2/2(Pref)
  PSS selector/1 -> PSS selector1/1
  Constant9/1 -> Matrix Multiply1/1
  Turbine & Regulators M2/2(Vf) -> Synchronous Machine pu Standard/2, Bus Creator/2, Scope23/1
  PID Controller2/1 -> Sum/2
  Constant11/1 -> Kalman Filter2/4
  "Phasor Measurement Unit (PMU, Three-Phase)4"/1 -> Scope39/1
  Bus Selector3/1 -> PID Controller1/1, Fcn2/1  "<Rotor speed deviation  dw (pu)>"
  Synchronous Machine pu Standard/1 -> Bus Selector2/1, Subtract/1, Kalman Filter/2, Turbine & Regulators M2/1(m)
  Constant1/1 -> Sum1/1
  Vref1 1/1 -> Sum2/1
  Fcn2/1 -> [B4], Scope6/1
  Bus Selector2/2 -> Display1/1, Scope5/1  "<Electrical power  Pe (pu)>"
  Three-Phase V-I Measurement8/1 -> Scope18/1
  Constant6/1 -> Kalman Filter1/3
  "Phasor Measurement Unit (PMU, Three-Phase)2"/1 -> Scope33/1
  Matrix Multiply1/1 -> Subtract1/2
  Fcn1/1 -> [B1], Scope2/1
  Three-Phase V-I Measurement7/1 -> Scope17/1
  Constant5/1 -> Matrix Multiply/1
  From2/1 -> "PMU (PLL-Based, Positive-Sequence)5"/1
  "PMU (PLL-Based, Positive-Sequence)3"/1 -> Scope55/1
  Constant4/1 -> Kalman Filter/5
  Rate Transition2/1 -> Bus Creator1/1
  Subtract/1 -> MATLAB Function/1(u)
  "Phasor Measurement Unit (PMU, Three-Phase)"/3 -> Scope29/1
  Three-Phase V-I Measurement5/1 -> "Phasor Measurement Unit (PMU, Three-Phase)3"/1, Scope15/1
  Constant7/1 -> Kalman Filter1/4
  PSS selector1/1 -> [PSS]
  Three-Phase V-I Measurement3/1 -> "PMU (PLL-Based, Positive-Sequence)2"/1, Scope12/1
  Bus Selector1/2 -> [B5], Display5/1, PLL5/1, Scope3/1, Scope3/2  "<Electrical power  Pe (pu)>"
  "PMU (PLL-Based, Positive-Sequence)5"/1 -> Scope59/1
  [FDIA] -> Sum2/3
  Kalman Filter2/1 -> Matrix Multiply2/2
  Fcn3/1 -> [B3], Scope4/1
  "PMU (PLL-Based, Positive-Sequence)6"/3 -> Scope60/3
  Turbine & Regulators M3/2(Vf) -> Synchronous Machine pu Standard2/2, Rate Transition5/1, Scope21/1
  Turbine & Regulators M3/1(Pm) -> Rate Transition4/1, Synchronous Machine pu Standard2/1
  MATLAB Function2/1(y) -> [B2], Scope19/1
  Synchronous Machine pu Standard2/1 -> Subtract2/1, Kalman Filter2/2, Bus Selector1/1, Turbine & Regulators M3/1(m)
  Constant2/1 -> Sum/1
  "PMU (PLL-Based, Positive-Sequence)8"/1 -> Scope57/1
  "Phasor Measurement Unit (PMU, Three-Phase)3"/1 -> Scope36/1
  "PMU (PLL-Based, Positive-Sequence)4"/1 -> Scope58/1
  "Power (3ph, Phasor)"/1 -> PLL2/1, Scope25/1
  "PMU (PLL-Based, Positive-Sequence)8"/3 -> Scope57/3
  "PMU (PLL-Based, Positive-Sequence)3"/3 -> Scope55/3
  Turbine & Regulators M1/2(Vf) -> Rate Transition3/1, Scope22/1, Synchronous Machine pu Standard1/2
  Bus Selector3/2 -> PLL4/1, [B7], Display3/1, Scope7/1  "<Electrical power  Pe (pu)>"
  PLL4/2 -> Display2/1
  Three-Phase V-I Measurement4/1 -> "Phasor Measurement Unit (PMU, Three-Phase)1"/1, Scope20/1, "Power (3ph, Phasor)1"/1
  PID Controller1/1 -> Sum2/2, Sum1/2
  "Phasor Measurement Unit (PMU, Three-Phase)"/2 -> Scope28/1
  Matrix Multiply/1 -> Subtract/2
  "Phasor Measurement Unit (PMU, Three-Phase)1"/2 -> Scope31/1
  Kalman Filter1/1 -> Matrix Multiply1/2
  "Power (3ph, Phasor)1"/1 -> Scope14/1
  "Phasor Measurement Unit (PMU, Three-Phase)"/1 -> Scope/1
  From3/1 -> "PMU (PLL-Based, Positive-Sequence)6"/1
  Three-Phase V-I Measurement3/2 -> Scope13/1
  Bus Selector2/1 -> Scope51/1, Fcn3/1  "<Rotor speed deviation  dw (pu)>"
  MATLAB Function1/1(y) -> [B9], Scope8/1
  "Phasor Measurement Unit (PMU, Three-Phase)1"/3 -> Scope32/1
  "Phasor Measurement Unit (PMU, Three-Phase)3"/3 -> Scope38/1
  Synchronous Machine pu Standard1/1 -> Subtract1/1, Kalman Filter1/2, Bus Selector3/1, Turbine & Regulators M1/1(m)
  "Phasor Measurement Unit (PMU, Three-Phase)2"/2 -> Scope35/1
  PLL/1 -> Scope43/1
  "PMU (PLL-Based, Positive-Sequence)7"/1 -> Scope56/1
  "Phasor Measurement Unit (PMU, Three-Phase)2"/3 -> Scope34/1
  PLL (3ph)/1 -> Scope47/1
  Bus Selector1/1 -> PID Controller2/1, Fcn1/1  "<Rotor speed deviation  dw (pu)>"
  Turbine & Regulators M1/1(Pm) -> Rate Transition2/1, Synchronous Machine pu Standard1/1
  "PMU (PLL-Based, Positive-Sequence)2"/2 -> Scope53/1
  Fcn4/1 -> [B8]
  Demux/1 -> [LAA]
  Demux/2 -> [FDIA]
  Inport/1 -> Demux/1
  [B1] -> Mux/1
  [B2] -> Mux/2
  [B3] -> output_mux/1, Mux/3  "frequency"
  [B4] -> Mux/4
  [B5] -> Mux/5
  Mux/1 -> Outport/1
  [B7] -> Mux/6
  [B9] -> Mux/8
  [B8] -> output_mux/2, Mux/7  "residue"
  output_mux/1 -> Outport1/1
  connections:
  Synchronous Machine pu Standard1/RConn3 -- Three-Phase Parallel RLC Load1/LConn3 -- Three-Phase Transformer (Two Windings)1/LConn3 -- Three-Phase V-I Measurement3/LConn3
  Synchronous Machine pu Standard/RConn3 -- Three-Phase Parallel RLC Load3/LConn3 -- Three-Phase Transformer (Two Windings)/LConn3 -- Three-Phase V-I Measurement9/LConn3
  Bus_2/RConn11 -- Three-Phase PI Section Line5/LConn2 -- Three-Phase V-I Measurement2/LConn2
  Three-Phase PI Section Line5/RConn2 -- Bus_3/RConn2 -- Three-Phase V-I Measurement4/LConn2
  Three-Phase Transformer (Two Windings)3/LConn1 -- Three-Phase Parallel RLC Load2/LConn1 -- Three-Phase V-I Measurement1/LConn1 -- Synchronous Machine pu Standard2/RConn1
  Three-Phase Series RLC Load10/LConn1 -- Bus_2/RConn3 -- Three-Phase Breaker2/RConn1
  Bus_2/LConn8 -- Three-Phase PI Section Line4/LConn2 -- Three-Phase V-I Measurement5/LConn2
  Three-Phase PI Section Line5/RConn3 -- Bus_3/RConn3 -- Three-Phase V-I Measurement4/LConn3
  Three-Phase PI Section Line4/RConn2 -- Bus_4/RConn5 -- Three-Phase V-I Measurement6/LConn2
  Bus_2/RConn12 -- Three-Phase PI Section Line5/LConn1 -- Three-Phase V-I Measurement2/LConn1
  Three-Phase Series RLC Load10/LConn2 -- Bus_2/RConn5 -- Three-Phase Breaker2/RConn2
  Three-Phase PI Section Line5/RConn1 -- Bus_3/RConn1 -- Three-Phase V-I Measurement4/LConn1
  Three-Phase PI Section Line18/RConn2 -- Bus_14/RConn2 -- Three-Phase V-I Measurement8/LConn2
  Three-Phase Transformer (Two Windings)/LConn2 -- Three-Phase Parallel RLC Load3/LConn2 -- Three-Phase V-I Measurement9/LConn2 -- Synchronous Machine pu Standard/RConn2
  Bus_13/RConn8 -- Three-Phase PI Section Line18/LConn2 -- Three-Phase V-I Measurement7/LConn2
  Bus_2/RConn10 -- Three-Phase PI Section Line5/LConn3 -- Three-Phase V-I Measurement2/LConn3
  Synchronous Machine pu Standard1/RConn1 -- Three-Phase Parallel RLC Load1/LConn1 -- Three-Phase Transformer (Two Windings)1/LConn1 -- Three-Phase V-I Measurement3/LConn1
  Three-Phase Breaker/RConn2 -- Three-Phase Breaker1/RConn2 -- Bus_3/RConn5
  Three-Phase PI Section Line4/RConn1 -- Bus_4/RConn4 -- Three-Phase V-I Measurement6/LConn1
  Synchronous Machine pu Standard1/RConn2 -- Three-Phase Parallel RLC Load1/LConn2 -- Three-Phase Transformer (Two Windings)1/LConn2 -- Three-Phase V-I Measurement3/LConn2
  Three-Phase PI Section Line18/RConn3 -- Bus_14/RConn3 -- Three-Phase V-I Measurement8/LConn3
  Three-Phase Breaker/RConn3 -- Three-Phase Breaker1/RConn3 -- Bus_3/RConn6
  Three-Phase Transformer (Two Windings)/LConn1 -- Three-Phase Parallel RLC Load3/LConn1 -- Three-Phase V-I Measurement9/LConn1 -- Synchronous Machine pu Standard/RConn1
  Three-Phase PI Section Line4/RConn3 -- Bus_4/RConn6 -- Three-Phase V-I Measurement6/LConn3
  Synchronous Machine pu Standard2/RConn3 -- Three-Phase Parallel RLC Load2/LConn3 -- Three-Phase Transformer (Two Windings)3/LConn3 -- Three-Phase V-I Measurement1/LConn3
  Bus_2/LConn9 -- Three-Phase PI Section Line4/LConn3 -- Three-Phase V-I Measurement5/LConn3
  Three-Phase V-I Measurement7/LConn1 -- Three-Phase PI Section Line18/LConn1 -- Bus_13/RConn9
  Synchronous Machine pu Standard2/RConn2 -- Three-Phase Parallel RLC Load2/LConn2 -- Three-Phase Transformer (Two Windings)3/LConn2 -- Three-Phase V-I Measurement1/LConn2
  Three-Phase Series RLC Load10/LConn3 -- Bus_2/RConn6 -- Three-Phase Breaker2/RConn3
  Three-Phase PI Section Line18/RConn1 -- Bus_14/RConn1 -- Three-Phase V-I Measurement8/LConn1
  Bus_2/LConn7 -- Three-Phase PI Section Line4/LConn1 -- Three-Phase V-I Measurement5/LConn1
  Three-Phase Breaker/RConn1 -- Three-Phase Breaker1/RConn1 -- Bus_3/RConn4
  Bus_13/RConn7 -- Three-Phase PI Section Line18/LConn3 -- Three-Phase V-I Measurement7/LConn3
  Bus_6/LConn3 -- Three-Phase Transformer (Two Windings)2/RConn3
  Bus_9/RConn3 -- Three-Phase PI Section Line11/RConn3
  Bus_9/LConn4 -- Three-Phase Series RLC Load11/LConn1
  Bus_6/RConn4 -- Three-Phase PI Section Line16/RConn1
  Three-Phase PI Section Line15/LConn3 -- Bus_12/RConn4
  Three-Phase PI Section Line12/LConn2 -- Bus_11/RConn5
  Three-Phase PI Section Line10/LConn2 -- Bus_9/RConn5
  Three-Phase Series RLC Load4/LConn2 -- Bus_6/RConn11
  Three-Phase PI Section Line12/LConn1 -- Bus_11/RConn6
  Bus_6/RConn8 -- Three-Phase PI Section Line17/LConn2
  Three-Phase Source/RConn2 -- Three-Phase Transformer (Two Windings)4/LConn2
  Bus_12/LConn3 -- Three-Phase Series RLC Load7/LConn3
  Three-Phase Series RLC Load3/LConn3 -- Bus_5/LConn1
  Bus_1/RConn2 -- Three-Phase PI Section Line/LConn2
  Three-Phase PI Section Line7/LConn1 -- Bus_7/LConn1
  Three-Phase PI Section Line13/LConn3 -- Bus_6/LConn6
  Bus_6/RConn5 -- Three-Phase PI Section Line16/RConn2
  Three-Phase Series RLC Load4/LConn3 -- Bus_6/RConn12
  Three-Phase PI Section Line7/LConn3 -- Bus_7/LConn3
  Three-Phase PI Section Line8/LConn3 -- Bus_7/RConn6
  Three-Phase PI Section Line7/LConn2 -- Bus_7/LConn2
  Three-Phase PI Section Line7/RConn1 -- Bus_4/LConn4
  Three-Phase Series RLC Load2/LConn3 -- Bus_4/RConn12
  Bus_11/LConn3 -- Three-Phase Series RLC Load6/LConn3
  Bus_5/RConn3 -- Three-Phase PI Section Line1/RConn3
  Bus_1/LConn2 -- Three-Phase Transformer (Two Windings)/RConn2
  Three-Phase Series RLC Load9/LConn1 -- Bus_9/RConn12
  Three-Phase PI Section Line13/RConn1 -- Bus_5/LConn4
  Three-Phase PI Section Line14/RConn1 -- Bus_6/RConn1
  Bus_7/RConn1 -- Three-Phase PI Section Line9/RConn1
  Bus_4/RConn3 -- Three-Phase PI Section Line3/RConn3
  Three-Phase PI Section Line9/LConn3 -- Bus_9/RConn9
  Bus_5/RConn4 -- Three-Phase PI Section Line2/RConn3
  Three-Phase Transformer (Two Windings)3/RConn3 -- Bus_3/RConn9
  Three-Phase Transformer (Two Windings)4/RConn1 -- Three-Phase V-I Measurement/RConn1
  Three-Phase PI Section Line11/LConn1 -- Bus_10/RConn6
  Bus_9/LConn5 -- Three-Phase Series RLC Load11/LConn2
  Three-Phase PI Section Line3/LConn1 -- Bus_5/RConn9
  Three-Phase Transformer (Two Windings)1/RConn1 -- Bus_2/RConn7
  Three-Phase Source/RConn3 -- Three-Phase Transformer (Two Windings)4/LConn3
  Three-Phase Series RLC Load2/LConn2 -- Bus_4/RConn11
  Bus_1/LConn3 -- Three-Phase Transformer (Two Windings)/RConn1
  Three-Phase Breaker2/LConn2 -- Three-Phase Series RLC Load1/LConn2
  Three-Phase PI Section Line8/RConn3 -- Three-Phase V-I Measurement/LConn3
  Bus_12/RConn1 -- Three-Phase PI Section Line14/LConn1
  Bus_4/RConn9 -- Three-Phase PI Section Line6/LConn3
  Bus_13/LConn1 -- Three-Phase Series RLC Load8/LConn1
  Bus_1/RConn4 -- Three-Phase PI Section Line1/LConn3
  Three-Phase Breaker2/LConn3 -- Three-Phase Series RLC Load1/LConn3
  Bus_4/RConn2 -- Three-Phase PI Section Line3/RConn2
  Three-Phase Series RLC Load3/LConn2 -- Bus_5/LConn2
  Three-Phase PI Section Line12/LConn3 -- Bus_11/RConn4
  Three-Phase PI Section Line13/LConn1 -- Bus_6/LConn4
  Bus_1/RConn3 -- Three-Phase PI Section Line/LConn3
  Three-Phase PI Section Line13/LConn2 -- Bus_6/LConn5
  Three-Phase Series RLC Load2/LConn1 -- Bus_4/RConn10
  Three-Phase PI Section Line2/LConn1 -- Bus_2/LConn6
  Bus_5/RConn5 -- Three-Phase PI Section Line2/RConn2
  Three-Phase PI Section Line13/RConn2 -- Bus_5/LConn5
  Three-Phase Series RLC Load12/LConn2 -- Bus_14/LConn2
  Bus_10/RConn3 -- Three-Phase PI Section Line12/RConn3
  Bus_13/RConn3 -- Three-Phase PI Section Line15/RConn3
  Three-Phase Transformer (Two Windings)4/RConn2 -- Three-Phase V-I Measurement/RConn2
  Bus_14/LConn1 -- Three-Phase Series RLC Load12/LConn1
  Three-Phase Transformer (Two Windings)3/RConn1 -- Bus_3/RConn7
  Three-Phase PI Section Line15/LConn1 -- Bus_12/RConn6
  Three-Phase Series RLC Load6/LConn2 -- Bus_11/LConn2
  Bus_12/RConn2 -- Three-Phase PI Section Line14/LConn2
  Three-Phase PI Section Line2/LConn2 -- Bus_2/LConn5
  Bus_4/RConn1 -- Three-Phase PI Section Line3/RConn1
  Bus_6/LConn2 -- Three-Phase Transformer (Two Windings)2/RConn2
  Three-Phase PI Section Line9/LConn1 -- Bus_9/RConn7
  Three-Phase PI Section Line14/RConn2 -- Bus_6/RConn2
  Bus_13/RConn2 -- Three-Phase PI Section Line15/RConn2
  Bus_11/RConn3 -- Three-Phase PI Section Line17/RConn3
  Three-Phase PI Section Line3/LConn3 -- Bus_5/RConn7
  Bus_11/RConn1 -- Three-Phase PI Section Line17/RConn1
  Three-Phase Breaker/LConn1 -- Three-Phase Series RLC Load14/LConn1
  Bus_9/LConn2 -- Three-Phase PI Section Line19/RConn2
  Three-Phase Series RLC Load9/LConn3 -- Bus_9/RConn10
  Three-Phase PI Section Line16/LConn1 -- Bus_13/RConn4
  Three-Phase Series RLC Load9/LConn2 -- Bus_9/RConn11
  Bus_9/LConn6 -- Three-Phase Series RLC Load11/LConn3
  Three-Phase Series RLC Load14/LConn2 -- Three-Phase Breaker/LConn2
  Bus_1/RConn1 -- Three-Phase PI Section Line/LConn1
  Bus_10/RConn1 -- Three-Phase PI Section Line12/RConn1
  Three-Phase PI Section Line8/RConn1 -- Three-Phase V-I Measurement/LConn1
  Bus_7/RConn2 -- Three-Phase PI Section Line9/RConn2
  Bus_12/LConn1 -- Three-Phase Series RLC Load7/LConn1
  Three-Phase PI Section Line10/LConn1 -- Bus_9/RConn4
  Bus_5/RConn6 -- Three-Phase PI Section Line2/RConn1
  Three-Phase PI Section Line14/RConn3 -- Bus_6/RConn3
  Three-Phase PI Section Line11/LConn2 -- Bus_10/RConn5
  Three-Phase Series RLC Load3/LConn1 -- Bus_5/LConn3
  Bus_1/RConn5 -- Three-Phase PI Section Line1/LConn2
  Three-Phase PI Section Line9/LConn2 -- Bus_9/RConn8
  Three-Phase Transformer (Two Windings)3/RConn2 -- Bus_3/RConn8
  Bus_4/RConn7 -- Three-Phase PI Section Line6/LConn1
  Three-Phase PI Section Line6/RConn2 -- Bus_3/LConn2
  Bus_2/LConn2 -- Three-Phase PI Section Line/RConn2
  Three-Phase Transformer (Two Windings)2/LConn2 -- Three-Phase Source1/RConn2
  Bus_12/RConn3 -- Three-Phase PI Section Line14/LConn3
  Three-Phase PI Section Line2/LConn3 -- Bus_2/LConn4
  Three-Phase PI Section Line19/LConn3 -- Bus_14/RConn6
  Bus_5/RConn1 -- Three-Phase PI Section Line1/RConn1
  Bus_13/LConn3 -- Three-Phase Series RLC Load8/LConn3
  Three-Phase PI Section Line16/LConn3 -- Bus_13/RConn6
  Bus_6/RConn9 -- Three-Phase PI Section Line17/LConn3
  Bus_6/RConn6 -- Three-Phase PI Section Line16/RConn3
  Bus_6/RConn7 -- Three-Phase PI Section Line17/LConn1
  Bus_4/LConn1 -- Three-Phase PI Section Line10/RConn1
  Three-Phase Breaker1/LConn2 -- Three-Phase Series RLC Load13/LConn2
  Three-Phase Source/RConn1 -- Three-Phase Transformer (Two Windings)4/LConn1
  Three-Phase PI Section Line10/LConn3 -- Bus_9/RConn6
  Three-Phase Transformer (Two Windings)2/LConn3 -- Three-Phase Source1/RConn3
  Bus_10/RConn2 -- Three-Phase PI Section Line12/RConn2
  Three-Phase PI Section Line11/LConn3 -- Bus_10/RConn4
  Bus_1/LConn1 -- Three-Phase Transformer (Two Windings)/RConn3
  Bus_11/RConn2 -- Three-Phase PI Section Line17/RConn2
  Three-Phase PI Section Line19/LConn2 -- Bus_14/RConn5
  Three-Phase PI Section Line8/LConn1 -- Bus_7/RConn4
  Bus_4/RConn8 -- Three-Phase PI Section Line6/LConn2
  Bus_5/RConn2 -- Three-Phase PI Section Line1/RConn2
  Three-Phase PI Section Line8/LConn2 -- Bus_7/RConn5
  Bus_12/LConn2 -- Three-Phase Series RLC Load7/LConn2
  Bus_1/RConn6 -- Three-Phase PI Section Line1/LConn1
  Bus_9/LConn1 -- Three-Phase PI Section Line19/RConn1
  Three-Phase Breaker2/LConn1 -- Three-Phase Series RLC Load1/LConn1
  Three-Phase PI Section Line7/RConn2 -- Bus_4/LConn5
  Bus_2/LConn3 -- Three-Phase PI Section Line/RConn3
  Bus_2/RConn9 -- Three-Phase Transformer (Two Windings)1/RConn3
  Bus_9/RConn2 -- Three-Phase PI Section Line11/RConn2
  Three-Phase PI Section Line3/LConn2 -- Bus_5/RConn8
  Three-Phase PI Section Line7/RConn3 -- Bus_4/LConn6
  Three-Phase Transformer (Two Windings)1/RConn2 -- Bus_2/RConn8
  Three-Phase Series RLC Load5/LConn1 -- Bus_10/LConn1
  Three-Phase Series RLC Load13/LConn3 -- Three-Phase Breaker1/LConn3
  Bus_4/LConn2 -- Three-Phase PI Section Line10/RConn2
  Three-Phase PI Section Line13/RConn3 -- Bus_5/LConn6
  Bus_6/LConn1 -- Three-Phase Transformer (Two Windings)2/RConn1
  Bus_11/LConn1 -- Three-Phase Series RLC Load6/LConn1
  Three-Phase Series RLC Load5/LConn2 -- Bus_10/LConn2
  Three-Phase Series RLC Load14/LConn3 -- Three-Phase Breaker/LConn3
  Three-Phase Series RLC Load4/LConn1 -- Bus_6/RConn10
  Three-Phase PI Section Line6/RConn3 -- Bus_3/LConn3
  Three-Phase PI Section Line16/LConn2 -- Bus_13/RConn5
  Bus_9/LConn3 -- Three-Phase PI Section Line19/RConn3
  Bus_9/RConn1 -- Three-Phase PI Section Line11/RConn1
  Three-Phase Breaker1/LConn1 -- Three-Phase Series RLC Load13/LConn1
  Three-Phase PI Section Line19/LConn1 -- Bus_14/RConn4
  Three-Phase Transformer (Two Windings)2/LConn1 -- Three-Phase Source1/RConn1
  Bus_2/LConn1 -- Three-Phase PI Section Line/RConn1
  Bus_13/LConn2 -- Three-Phase Series RLC Load8/LConn2
  Three-Phase Series RLC Load5/LConn3 -- Bus_10/LConn3
  Bus_14/LConn3 -- Three-Phase Series RLC Load12/LConn3
  Three-Phase PI Section Line6/RConn1 -- Bus_3/LConn1
  Bus_7/RConn3 -- Three-Phase PI Section Line9/RConn3
  Bus_13/RConn1 -- Three-Phase PI Section Line15/RConn1
  Three-Phase V-I Measurement/LConn2 -- Three-Phase PI Section Line8/RConn2
  Bus_4/LConn3 -- Three-Phase PI Section Line10/RConn3
  Three-Phase PI Section Line15/LConn2 -- Bus_12/RConn5
  Three-Phase Transformer (Two Windings)4/RConn3 -- Three-Phase V-I Measurement/RConn3
